simulink model "GPC"  (R2020b)
settings: Solver=VariableStepAuto  StartTime=0.0  StopTime=30  RelTol=1e-3
undefined symbols (not defined in the file): C_siso, C_siso_2, KE_siso, KE_siso_2, KF_siso, KF_siso_2, Kr_siso, Kr_siso_2
libraries: cstblocks x2
settings Model: Creator=LACER_GMG  LastModifiedBy=GMG
settings SolverCC: AlgebraicLoopSolver=LineSearch

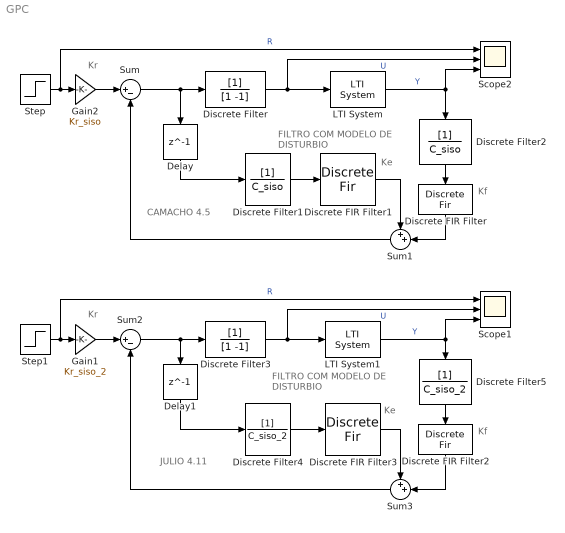
== system GPC ==
  note: Ke
  note: FILTRO COM MODELO
      | DE DISTURBIO
  note: JULIO 4.11
  note: CAMACHO 4.5
  note: Kf
  note: Kr
  note: Kr
  note: Ke
  note: Kf
  note: FILTRO COM MODELO
      | DE DISTURBIO
  Delay : Delay  DelayLength=1  InitialCondition=0
  Delay1 : Delay  DelayLength=1  InitialCondition=0
  Discrete FIR Filter : DiscreteFir  Coefficients=KF_siso  SampleTime=1
  Discrete FIR Filter1 : DiscreteFir  Coefficients=KE_siso  SampleTime=1
  Discrete FIR Filter2 : DiscreteFir  Coefficients=KF_siso_2  SampleTime=1
  Discrete FIR Filter3 : DiscreteFir  Coefficients=KE_siso_2  SampleTime=1
  Discrete Filter : DiscreteFilter  Denominator=[1 -1]  SampleTime=1
  Discrete Filter1 : DiscreteFilter  Denominator=C_siso  SampleTime=1
  Discrete Filter2 : DiscreteFilter  Denominator=C_siso  SampleTime=1
  Discrete Filter3 : DiscreteFilter  Denominator=[1 -1]  SampleTime=1
  Discrete Filter4 : DiscreteFilter  Denominator=C_siso_2  SampleTime=1
  Discrete Filter5 : DiscreteFilter  Denominator=C_siso_2  SampleTime=1
  Gain1 : Gain  Gain=Kr_siso_2
  Gain2 : Gain  Gain=Kr_siso
  LTI System : cstblocks/LTI System  sys=P_siso  IC=[]
  LTI System1 : cstblocks/LTI System  sys=P_siso_2  IC=[]
  Scope1 : Scope  NumInputPorts=3
  Scope2 : Scope  NumInputPorts=3
  Step : Step  SampleTime=1
  Step1 : Step  SampleTime=1
  Sum : Sum  Inputs=|+-
  Sum1 : Sum  Inputs=++|
  Sum2 : Sum  Inputs=|+-
  Sum3 : Sum  Inputs=++|
  wires:
  Step/1 -> Scope2/1, Gain2/1  "R"
  Sum/1 -> Discrete Filter/1, Delay/1
  Discrete Filter/1 -> Scope2/2, LTI System/1  "U"
  Sum1/1 -> Sum/2
  Gain2/1 -> Sum/1
  Discrete FIR Filter/1 -> Sum1/2
  Discrete FIR Filter1/1 -> Sum1/1
  Delay/1 -> Discrete Filter1/1
  Discrete Filter1/1 -> Discrete FIR Filter1/1
  Discrete Filter2/1 -> Discrete FIR Filter/1
  Sum3/1 -> Sum2/2
  Discrete Filter4/1 -> Discrete FIR Filter3/1
  Discrete FIR Filter3/1 -> Sum3/1
  Discrete FIR Filter2/1 -> Sum3/2
  Discrete Filter3/1 -> Scope1/2, LTI System1/1  "U"
  Delay1/1 -> Discrete Filter4/1
  Discrete Filter5/1 -> Discrete FIR Filter2/1
  Step1/1 -> Scope1/1, Gain1/1  "R"
  Sum2/1 -> Discrete Filter3/1, Delay1/1
  LTI System1/1 -> Discrete Filter5/1, Scope1/3  "Y"
  Gain1/1 -> Sum2/1
  LTI System/1 -> Discrete Filter2/1, Scope2/3  "Y"
